simulink model "testpso"  (R2021a)
settings: Solver=FixedStepAuto  StartTime=0.0  StopTime=30  RelTol=1e-3
undefined symbols (not defined in the file or in its folder): kk
libraries: pid_lib x1
settings Model: Creator=uddin  LastModifiedBy=uddin
settings DataIOCC: SaveFormat=Array
settings OptimizationCC: OptimizeBlockIOStorage=off  BufferReuse=off  OptimizeDataStoreBuffers=off  BusAssignmentInplaceUpdate=off
settings DebuggingCC: SFUnexpectedBacktrackingDiag=warning  SFNoUnconditionalDefaultTransitionDiag=warning
settings RTWCC: GenerateReport=on  BuildConfiguration=Debug  LaunchReport=on
settings CodeAppCC: ForceParamTrailComments=on  MATLABSourceComments=on  EnableCustomComments=on
settings GRTTargetCC: CombineSignalStateStructs=on  CodeInterfacePackaging=Reusable function  SupportVariableSizeSignals=on  GenerateAllocFcn=on  MultiInstanceErrorCode=Warning

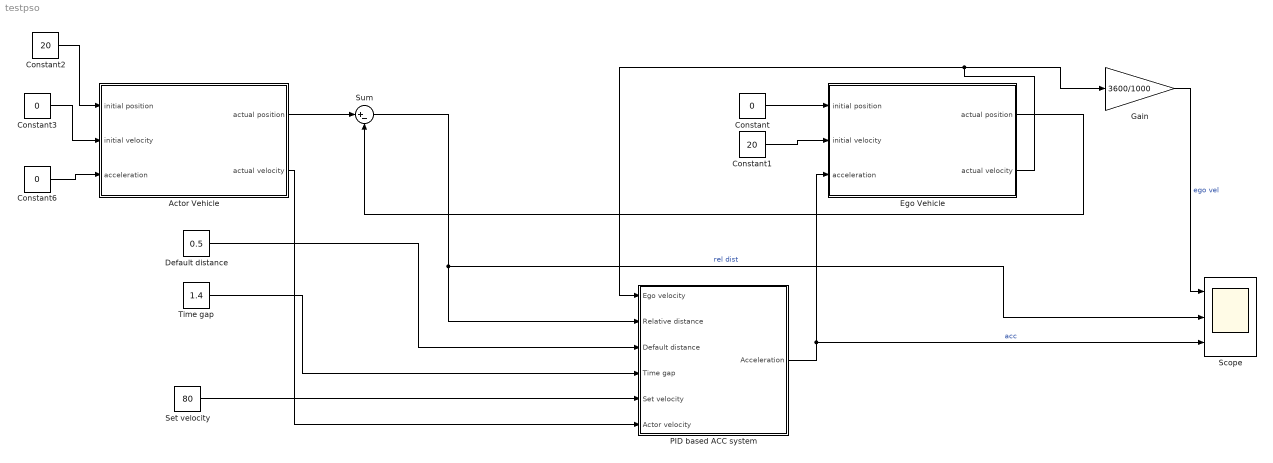
== system testpso ==
  Actor Vehicle : Subsystem
  Constant : Constant  Value=0  SampleTime=.1
  Constant1 : Constant  Value=20  SampleTime=.1
  Constant2 : Constant  Value=20  SampleTime=.1
  Constant3 : Constant  Value=0  SampleTime=.1
  Constant6 : Constant  Value=0  SampleTime=.1
  Default distance : Constant  Value=0.5  SampleTime=.1
  Ego Vehicle : Subsystem
  Gain : Gain  Gain=3600/1000
  PID based ACC system : Subsystem
  Scope : Scope  NumInputPorts=3
  Set velocity : Constant  Value=80  SampleTime=.1
  Sum : Sum  Inputs=|+-
  Time gap : Constant  Value=1.4  SampleTime=.1
  wires:
  Actor Vehicle/2(actual velocity) -> PID based ACC system/6(Actor velocity)
  PID based ACC system/1(Acceleration) -> Ego Vehicle/3(acceleration), Scope/3  "acc"
  Set velocity/1 -> PID based ACC system/5(Set velocity)
  Gain/1 -> Scope/1  "ego vel"
  Time gap/1 -> PID based ACC system/4(Time gap)
  Default distance/1 -> PID based ACC system/3(Default distance)
  Constant2/1 -> Actor Vehicle/1(initial position)
  Constant/1 -> Ego Vehicle/1(initial position)
  Sum/1 -> PID based ACC system/2(Relative distance), Scope/2  "rel dist"
  Constant6/1 -> Actor Vehicle/3(acceleration)
  Constant3/1 -> Actor Vehicle/2(initial velocity)
  Ego Vehicle/2(actual velocity) -> PID based ACC system/1(Ego velocity), Gain/1
  Constant1/1 -> Ego Vehicle/2(initial velocity)
  Ego Vehicle/1(actual position) -> Sum/2
  Actor Vehicle/1(actual position) -> Sum/1

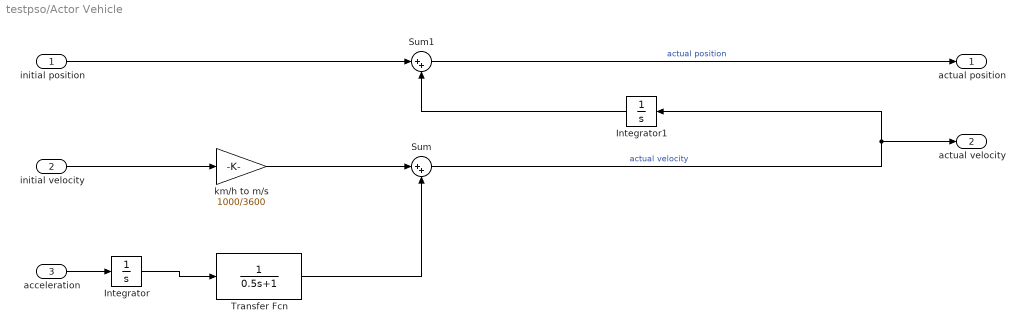
== system testpso/Actor Vehicle ==
  initial position : Inport
  initial velocity : Inport  Port=2
  acceleration : Inport  Port=3
  Integrator : Integrator
  Integrator1 : Integrator
  Sum : Sum  Inputs=|++
  Sum1 : Sum  Inputs=|++
  Transfer Fcn : TransferFcn  Denominator=[0.5 1]
  km/h to m/s : Gain  Gain=1000/3600
  actual position : Outport
  actual velocity : Outport  Port=2
  wires:
  km/h to m/s/1 -> Sum/1
  initial velocity/1 -> km/h to m/s/1
  Transfer Fcn/1 -> Sum/2
  Integrator/1 -> Transfer Fcn/1
  Integrator1/1 -> Sum1/2
  initial position/1 -> Sum1/1
  acceleration/1 -> Integrator/1
  Sum/1 -> Integrator1/1, actual velocity/1  "actual velocity"
  Sum1/1 -> actual position/1  "actual position"

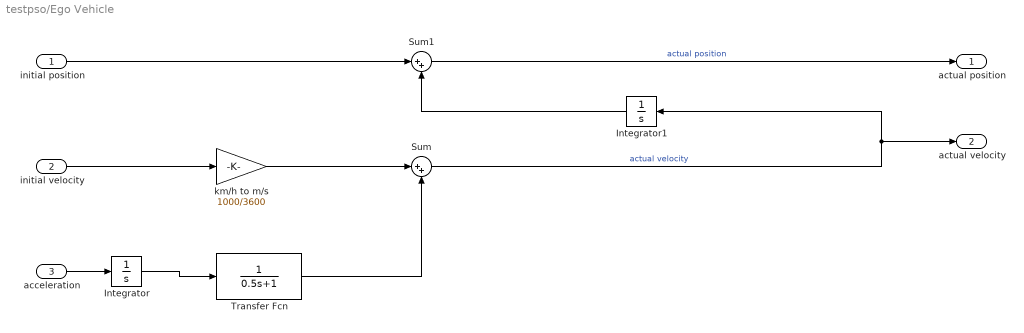
== system testpso/Ego Vehicle ==
  initial position : Inport
  initial velocity : Inport  Port=2
  acceleration : Inport  Port=3
  Integrator : Integrator
  Integrator1 : Integrator
  Sum : Sum  Inputs=|++
  Sum1 : Sum  Inputs=|++
  Transfer Fcn : TransferFcn  Denominator=[0.5 1]
  km/h to m/s : Gain  Gain=1000/3600
  actual position : Outport
  actual velocity : Outport  Port=2
  wires:
  Sum1/1 -> actual position/1  "actual position"
  Sum/1 -> actual velocity/1, Integrator1/1  "actual velocity"
  acceleration/1 -> Integrator/1
  initial position/1 -> Sum1/1
  Integrator1/1 -> Sum1/2
  Integrator/1 -> Transfer Fcn/1
  Transfer Fcn/1 -> Sum/2
  initial velocity/1 -> km/h to m/s/1
  km/h to m/s/1 -> Sum/1

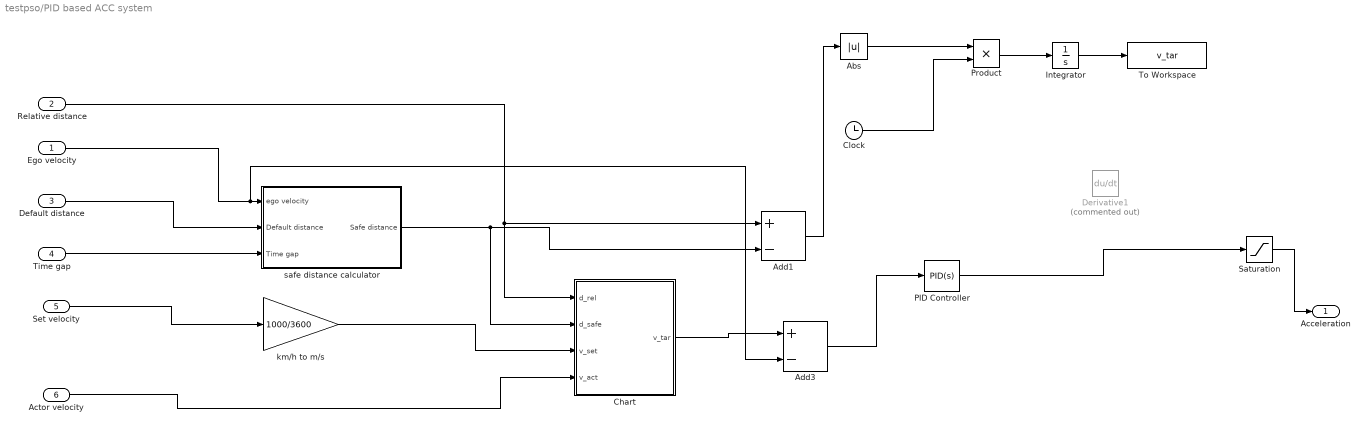
== system testpso/PID based ACC system ==
  Ego velocity : Inport
  Relative distance : Inport  Port=2
  Default distance : Inport  Port=3
  Time gap : Inport  Port=4
  Set velocity : Inport  Port=5
  Actor velocity : Inport  Port=6
  Abs : Abs
  Add1 : Sum  Inputs=+-
  Add3 : Sum  Inputs=+-
  Chart : Stateflow chart  TreatAsAtomicUnit=on
  Clock : Clock
  Derivative1 : Derivative  Commented=on
  Integrator : Integrator
  PID Controller : pid_lib/PID Controller  Controller=PID  Form=Parallel  TimeDomain=Continuous-time  UseExternalTs=off  SampleTime=-1  IntegratorMethod=Forward Euler  FilterMethod=Forward Euler  ControllerParametersSource=internal  P=kk(1)  I=kk(2)  D=kk(3)  UseFilter=on  N=1  TunerSelectOption=Transfer Function Based (PID Tuner App)  InitialConditionSource=internal  InitialConditionForIntegrator=0  InitialConditionForFilter=0  DifferentiatorICPrevScaledInput=0  ExternalReset=none  TrackingMode=off  Kt=1  LimitOutput=off  SatLimitsSource=internal  UpperSaturationLimit=inf  LowerSaturationLimit=-inf  LinearizeAsGain=on  AntiWindupMode=none  Kb=1  POutMin=[]  POutMax=[]  IOutMin=[]  IOutMax=[]  DOutMin=[]  DOutMax=[]  NOutMin=[]  NOutMax=[]  SumOutMin=[]  SumOutMax=[]  SaturationOutMin=[]  SaturationOutMax=[]  PParamMin=[]  PParamMax=[]  IParamMin=[]  IParamMax=[]  DParamMin=[]  DParamMax=[]  NParamMin=[]  NParamMax=[]  KbParamMin=[]  KbParamMax=[]  KtParamMin=[]  KtParamMax=[]  KbOutMin=[]  KbOutMax=[]  KtOutMin=[]  KtOutMax=[]  IntegratorOutMin=[]  IntegratorOutMax=[]  FilterOutMin=[]  FilterOutMax=[]  SumI1OutMin=[]  SumI1OutMax=[]  SumI2OutMin=[]  SumI2OutMax=[]  SumI3OutMin=[]  SumI3OutMax=[]  SumI4OutMin=[]  SumI4OutMax=[]  SumDOutMin=[]  SumDOutMax=[]  DifferentiatorOutMin=[]  DifferentiatorOutMax=[]  FilterDiffOutCoefMin=[]  FilterDiffOutCoefMax=[]  ReciprocalOutMin=[]  ReciprocalOutMax=[]  SumDenOutMin=[]  SumDenOutMax=[]  SumNumOutMin=[]  SumNumOutMax=[]  DivideOutMin=[]  DivideOutMax=[]  UdiffTsProdOutMin=[]  UdiffTsProdOutMax=[]  NTsProdOutMin=[]  NTsProdOutMax=[]  UintegralTsProdOutMin=[]  UintegralTsProdOutMax=[]  UngainTsProdOutMin=[]  UngainTsProdOutMax=[]  IntegratorContinuousStateAttributes=''  IntegratorStateMustResolveToSignalObject=off  IntegratorRTWStateStorageClass=Auto  FilterContinuousStateAttributes=''  FilterStateMustResolveToSignalObject=off  FilterRTWStateStorageClass=Auto  ParallelPVariant=InternalParameters  IdealPVariant=Disabled  IVariant=InternalParameters  DVariant=InternalParameters  IntegratorVariant=Continuous  SatVariant=Disabled  AWVariant=Passthrough  PCopyVariant=Disabled  TRVariant=Disabled  FdbkBlocksVariant=Forward  IdealPFdbkVariant=Disabled  SatFdbkVariant=Disabled  DerivativeFilterVariant=ContFilter  NVariant=InternalParameters  NCopyVariant=Disabled  FilterICVariant=InternalICsFilter  IntegratorICVariant=InternalICs  ExternalResetVariant=Disabled  TRSumVariant=Passthrough  SumFdbkVariant=Disabled  SumVariant=Sum_PID  TsampFilterVariant=InternalTs  TsampNgainVariant=Passthrough  TsampIntegralVariant=Passthrough  ExternalSaturationOutDataTypeStr=Inherit: Same as second input
  Product : Product
  Saturation : Saturate  UpperLimit=2  LowerLimit=-3  LinearizeAsGain=off
  To Workspace : ToWorkspace  VariableName=v_tar  SampleTime=-1
      settings: Save2DSignal=2-D array (concatenate along first dimension)
  km/h to m/s : Gain  Gain=1000/3600
  safe distance calculator : Subsystem
  Acceleration : Outport
  wires:
  Default distance/1 -> safe distance calculator/2(Default distance)
  Set velocity/1 -> km/h to m/s/1
  Time gap/1 -> safe distance calculator/3(Time gap)
  Ego velocity/1 -> Add3/2, safe distance calculator/1(ego velocity)
  safe distance calculator/1(Safe distance) -> Add1/2, Chart/2(d_safe)
  Relative distance/1 -> Chart/1(d_rel), Add1/1
  km/h to m/s/1 -> Chart/3(v_set)
  Actor velocity/1 -> Chart/4(v_act)
  Saturation/1 -> Acceleration/1
  Chart/1(v_tar) -> Add3/1
  Clock/1 -> Product/2
  Product/1 -> Integrator/1
  Integrator/1 -> To Workspace/1
  Add1/1 -> Abs/1
  Abs/1 -> Product/1
  Add3/1 -> PID Controller/1
  PID Controller/1 -> Saturation/1

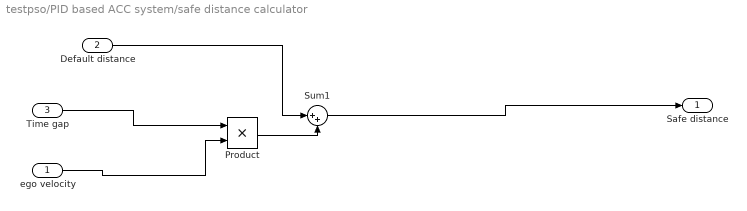
== system testpso/PID based ACC system/safe distance calculator ==
  ego velocity : Inport
  Default distance : Inport  Port=2
  Time gap : Inport  Port=3
  Product : Product
  Sum1 : Sum  Inputs=|++
  Safe distance : Outport
  wires:
  Product/1 -> Sum1/2
  Sum1/1 -> Safe distance/1
  Time gap/1 -> Product/1
  Default distance/1 -> Sum1/1
  ego velocity/1 -> Product/2

== stateflow chart testpso/PID based ACC system/Chart ==
  (default) -> (junction 7)
  (junction 7) -> (junction 8) [order 1] : [d_rel>d_safe]
  (junction 7) -> (junction 9) [order 2] : {v_tar=v_act;}
  (junction 8) -> (junction 10) : {v_tar=v_set;}
  (junction 10) -> (junction 9)
  (junction 9) -> (junction 11)
  data: d_rel input; d_safe input; v_set input; v_act input; v_tar output
